simulink model "MultirotorSimPx4v1_8TuningAttitudeDisc"  (R2020b)
settings: Solver=VariableStepAuto  StartTime=0.0  StopTime=Simulation.T_END  MaxStep=Simulation.TS_MAX  RelTol=1e-3  EnableMultiTasking=on
PreLoadFcn:
  | % InitializeParameters;
undefined symbols (not defined in the file): Initial, Simulation, Uav
libraries: QuaternionLibrary x17, simulink_extras x4
(part 7 of 7)

== matlab function MultirotorSimPx4v1_8TuningAttitudeDisc/Sensor Model/Accelerometer1/Quaternion to Rotation Matrix/MATLAB Function ==
  data: q input; R output
function R = QuatToRot( q )
%QUATTOROT Convert quaternion to rotation matrix
%   Written by:    J.X.J. Bannwarth, 2017/03/27
%   Last modified: J.X.J. Bannwarth, 2018/12/11
    W = q(1);
    X = q(2);
    Y = q(3);
    Z = q(4);
    
    xx = X * X;
    xy = X * Y;
    xz = X * Z;
    xw = X * W;

    yy = Y * Y;
    yz = Y * Z;
    yw = Y * W;
    
    zz = Z * Z;
    zw = Z * W;

    m00 = 1 - 2 * ( yy + zz );
    m01 =     2 * ( xy - zw );
    m02 =     2 * ( xz + yw );

    m10 =     2 * ( xy + zw );
    m11 = 1 - 2 * ( xx + zz );
    m12 =     2 * ( yz - xw );

    m20 =     2 * ( xz - yw );
    m21 =     2 * ( yz + xw );
    m22 = 1 - 2 * ( xx + yy );
    
    R = [m00 m01 m02;
         m10 m11 m12;
         m20 m21 m22];   
end

== matlab function MultirotorSimPx4v1_8TuningAttitudeDisc/Quadrotor Quaternion Model/Equations of motion ==
  data: VBody input; VBodyDot output; nuBody input; Q input; TBody input size=3; tauBody input size=3; F_D input size=3; M_D input size=3; time input; nuBodyDot output; Uav parameter; xiDDot output; Simulation parameter
function [VBodyDot, nuBodyDot, xiDDot] = QuadrotorQuaternionModel(...
    VBody, nuBody, Q, TBody, tauBody, F_D, M_D, time, Uav, Simulation)
%#codegen

%% Handle 2D pitch test
if isfield( Uav, 'PITCH_ONLY') && Uav.PITCH_ONLY
    tauBody = [0; 1; 0] .* tauBody;
    M_D = [0; 1; 0] .* M_D;
end

if isfield( Simulation, 'T_START_STEP') && ( time < Simulation.T_START_STEP )
    tauBody = [0; 0; 0] .* tauBody;
    M_D = [0; 0; 0] .* M_D;
end

%% Moments and Forces
% Body frame accelerations
VBodyDot  = (1/Uav.M) * (Q'*Uav.G + TBody - cross(nuBody, Uav.M*VBody) + F_D);
nuBodyDot = Uav.I \ (tauBody - cross(nuBody, Uav.I*nuBody) + M_D);

% Inertial frame accelerations
xiDDot = (1/Uav.M)*(Uav.G + Q*(TBody + F_D));
% etaDDot = WInvertDot*nuBody + WInvert*nuBodyDot;

% Check centripetal force in inertial frame
% F_C = R*cross(nuBody,m*VBody);

if Uav.PITCH_ONLY
    xiDDot = [1; 1; 0] .* xiDDot;
end

end

== matlab function MultirotorSimPx4v1_8TuningAttitudeDisc/L2 norm ==
  data: u input; y output
function y = l2norm( u )
    y = sqrt( dot(u, u) );
end

== matlab function MultirotorSimPx4v1_8TuningAttitudeDisc/Applied wind speed/Relative velocity ==
  data: nuBody input; Uav parameter; VMotorRelBody output
function VMotorRelBody = relativeMotorVelocity( nuBody , Uav )
%#codegen
    VMotorRelBody = cross( nuBody, Uav.L_VEC );
end

== matlab function MultirotorSimPx4v1_8TuningAttitudeDisc/Applied wind speed/Compute V_app2 ==
  data: Q input; UBody output; U input size=3
function UBody = computeUBody(Q, U)
%#codegen

% Rotation matrix from Wind frame to Inertial frame
% Wind frame SEU, inertial frame NED
R_U = [1,  0, 0;
       0, -1, 0;
       0,  0, 1];
   
UBody = Q' * R_U * U;

== matlab function MultirotorSimPx4v1_8TuningAttitudeDisc/Compute Sph ==
  data: in input; beta output; alpha output; R output
function [beta, alpha, R] = computeSph(in)
%#codegen

% Convert from polar to spherical coordinates
[ beta, alpha, R ] = cart2sph( in(1), in(2), in(3) );

== matlab function MultirotorSimPx4v1_8TuningAttitudeDisc/Sensor Model/Global reprojection/map_projection_reproject ==
  data: x input; y input; lat output; lon output; LAT0 parameter; LON0 parameter
function [ lat, lon ] = map_projection_reproject( x, y, LAT0, LON0)
%#codegen
%MAP_PROJECTION_REPROJECT
    M_DEG_TO_RAD = 0.017453292519943295;
	ref.lat_rad = LAT0 * M_DEG_TO_RAD;
	ref.lon_rad = LON0 * M_DEG_TO_RAD;
	ref.sin_lat = 0;
	ref.cos_lat = 0; 
    ref.sin_lat = sin(ref.lat_rad);
    ref.cos_lat = cos(ref.lat_rad);
    
    CONSTANTS_RADIUS_OF_EARTH = 6371000;
    M_PI = 3.14159265358979323846;

    x_rad = x / CONSTANTS_RADIUS_OF_EARTH;
    y_rad = y / CONSTANTS_RADIUS_OF_EARTH;
    c = sqrt(x_rad * x_rad + y_rad * y_rad);
    
    sin_c = sin(c);
    cos_c = cos(c);

    if (abs(c) > eps)
        lat_rad = asin(cos_c * ref.sin_lat + (x_rad * sin_c * ref.cos_lat) / c);
        lon_rad = (ref.lon_rad + atan2(y_rad * sin_c, c * ref.cos_lat * cos_c - x_rad * ref.sin_lat * sin_c));
    else
        lat_rad = ref.lat_rad;
        lon_rad = ref.lon_rad;
    end

    lat = lat_rad * 180.0 / M_PI;
    lon = lon_rad * 180.0 / M_PI;
end
